simulink model "SPC_3states"  (R2019b)
settings: Solver=VariableStepAuto  StartTime=0.0  StopTime=1500  RelTol=1e-3
values from neighbouring files (symbols this model uses):
  tau1 = 15    [SmithControl.m]    (also in TimeDelayParameters.m; positivity_matrix.m)
  tau2 = 20    [SmithControl.m]    (also in TimeDelayParameters.m = 30; positivity_matrix.m = 30)
  th1 = 0.85    [AP_TimeDelay.m]    (also in SmithControl.m; TimeDelayParameters.m = 0.32; positivity_matrix.m; rscale.m)
  th2 = 50    [AP_TimeDelay.m]    (also in SmithControl.m; TimeDelayParameters.m; positivity_matrix.m; rscale.m)
  th3 = 60    [AP_TimeDelay.m]    (also in SmithControl.m; TimeDelayParameters.m = 70; positivity_matrix.m; rscale.m)
  th4 = 5    [AP_TimeDelay.m]    (also in SmithControl.m; TimeDelayParameters.m = 2.7; positivity_matrix.m; rscale.m)
  th5 = 20    [AP_TimeDelay.m]    (also in SmithControl.m; TimeDelayParameters.m = 22; positivity_matrix.m; rscale.m)
settings Model: Creator=akshita_jain  LastModifiedBy=akshita_jain

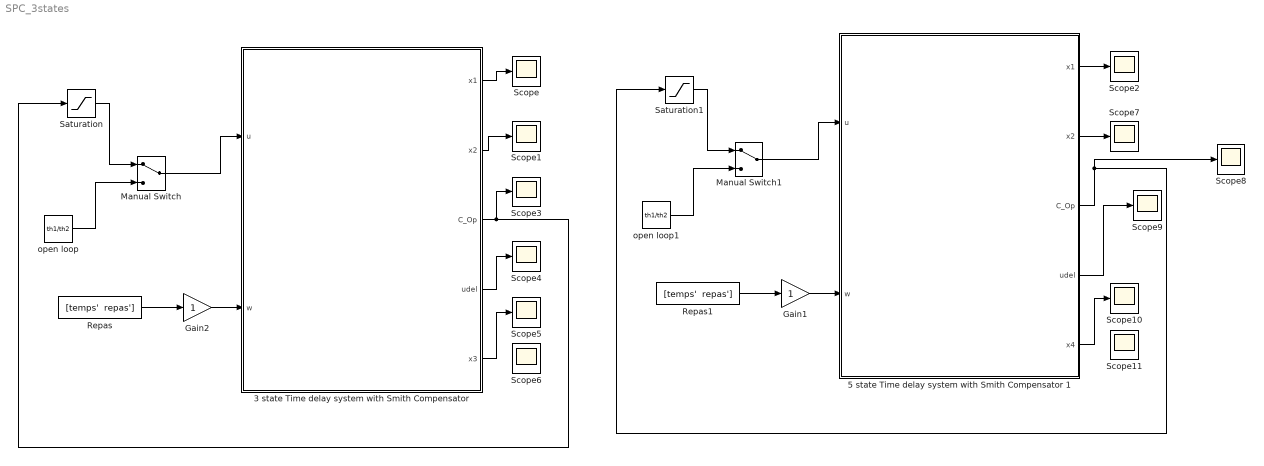
== system SPC_3states ==
  "3 state Time delay system with Smith Compensator " : Subsystem
  5 state Time delay system with Smith Compensator 1 : Subsystem
  Gain1 : Gain
  Gain2 : Gain
  Manual Switch : ManualSwitch
  Manual Switch1 : ManualSwitch
  Repas : FromWorkspace  VariableName="[temps'  repas']"  SampleTime=0
  Repas1 : FromWorkspace  VariableName="[temps'  repas']"  SampleTime=0
  Saturation : Saturate  UpperLimit=2  LowerLimit=0
  Saturation1 : Saturate  UpperLimit=2  LowerLimit=0
  Scope{,1..11} (12 alike) : Scope
  open loop : Constant  Value=th1/th2
  open loop1 : Constant  Value=th1/th2
  wires:
  "3 state Time delay system with Smith Compensator "/1(x1) -> Scope/1
  "3 state Time delay system with Smith Compensator "/3(C_Op) -> Scope3/1, Saturation/1
  "3 state Time delay system with Smith Compensator "/4(udel) -> Scope4/1
  "3 state Time delay system with Smith Compensator "/2(x2) -> Scope1/1
  Gain2/1 -> "3 state Time delay system with Smith Compensator "/2(w)
  Manual Switch/1 -> "3 state Time delay system with Smith Compensator "/1(u)
  Repas/1 -> Gain2/1
  open loop/1 -> Manual Switch/2
  Saturation/1 -> Manual Switch/1
  "3 state Time delay system with Smith Compensator "/5(x3) -> Scope5/1
  5 state Time delay system with Smith Compensator 1/1(x1) -> Scope2/1
  5 state Time delay system with Smith Compensator 1/4(udel) -> Scope9/1
  5 state Time delay system with Smith Compensator 1/2(x2) -> Scope7/1
  Gain1/1 -> 5 state Time delay system with Smith Compensator 1/2(w)
  Manual Switch1/1 -> 5 state Time delay system with Smith Compensator 1/1(u)
  open loop1/1 -> Manual Switch1/2
  Saturation1/1 -> Manual Switch1/1
  Repas1/1 -> Gain1/1
  5 state Time delay system with Smith Compensator 1/5(x4) -> Scope10/1
  5 state Time delay system with Smith Compensator 1/3(C_Op) -> Scope8/1, Saturation1/1

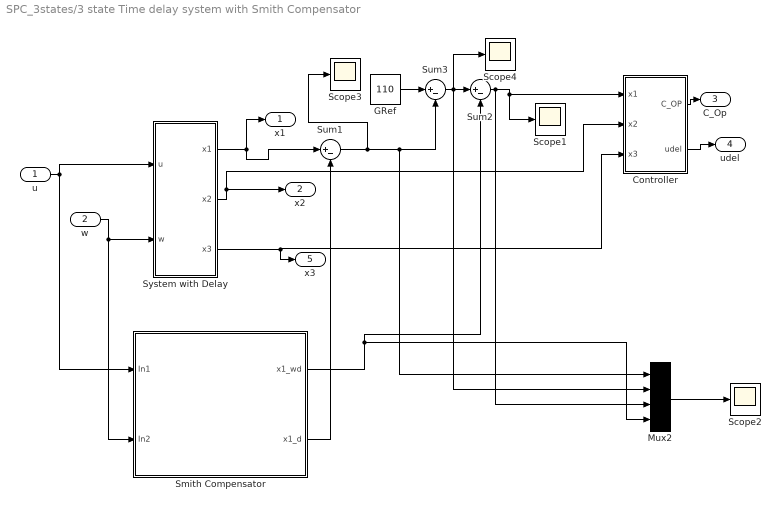
== system SPC_3states/3 state Time delay system with Smith Compensator  ==
  u : Inport
  w : Inport  Port=2
  "Controller " : Subsystem
  GRef : Constant  Value=110
  Mux2 : Mux
  Scope{1..4} (4 alike) : Scope
  Smith Compensator : Subsystem
  Sum1 : Sum  Inputs=|+-
  Sum2 : Sum  Inputs=|+-
  Sum3 : Sum  Inputs=|+-
  System with Delay : Subsystem
  x1 : Outport
  x2 : Outport  Port=2
  C_Op : Outport  Port=3
  udel : Outport  Port=4
  x3 : Outport  Port=5
  wires:
  u/1 -> Smith Compensator/1(In1), System with Delay/1(u)
  w/1 -> Smith Compensator/2(In2), System with Delay/2(w)
  System with Delay/1(x1) -> x1/1, Sum1/1
  Smith Compensator/2(x1_d) -> Sum1/2
  Sum1/1 -> Scope3/1, Mux2/1, Sum3/2
  Smith Compensator/1(x1_wd) -> Sum2/2, Mux2/4
  Sum2/1 -> Mux2/3, Scope1/1, "Controller "/1(x1)
  GRef/1 -> Sum3/1
  System with Delay/2(x2) -> "Controller "/2(x2), x2/1
  "Controller "/1(C_OP) -> C_Op/1
  "Controller "/2(udel) -> udel/1
  Mux2/1 -> Scope2/1
  Sum3/1 -> Scope4/1, Mux2/2, Sum2/1
  System with Delay/3(x3) -> "Controller "/3(x3), x3/1

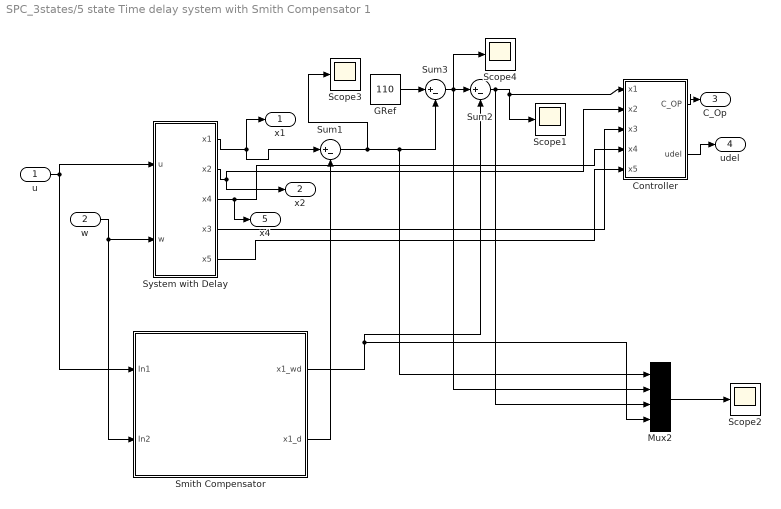
== system SPC_3states/5 state Time delay system with Smith Compensator 1 ==
  u : Inport
  w : Inport  Port=2
  "Controller " : Subsystem
  GRef : Constant  Value=110
  Mux2 : Mux
  Scope{1..4} (4 alike) : Scope
  Smith Compensator : Subsystem
  Sum1 : Sum  Inputs=|+-
  Sum2 : Sum  Inputs=|+-
  Sum3 : Sum  Inputs=|+-
  System with Delay : Subsystem
  x1 : Outport
  x2 : Outport  Port=2
  C_Op : Outport  Port=3
  udel : Outport  Port=4
  x4 : Outport  Port=5
  wires:
  u/1 -> Smith Compensator/1(In1), System with Delay/1(u)
  w/1 -> Smith Compensator/2(In2), System with Delay/2(w)
  System with Delay/1(x1) -> x1/1, Sum1/1
  Smith Compensator/2(x1_d) -> Sum1/2
  Sum1/1 -> Scope3/1, Mux2/1, Sum3/2
  Smith Compensator/1(x1_wd) -> Sum2/2, Mux2/4
  Sum2/1 -> Mux2/3, Scope1/1, "Controller "/1(x1)
  GRef/1 -> Sum3/1
  System with Delay/2(x2) -> x2/1, "Controller "/2(x2)
  "Controller "/1(C_OP) -> C_Op/1
  "Controller "/2(udel) -> udel/1
  Mux2/1 -> Scope2/1
  Sum3/1 -> Scope4/1, Mux2/2, Sum2/1
  System with Delay/4(x3) -> "Controller "/3(x3)
  System with Delay/3(x4) -> x4/1, "Controller "/4(x4)
  System with Delay/5(x5) -> "Controller "/5(x5)

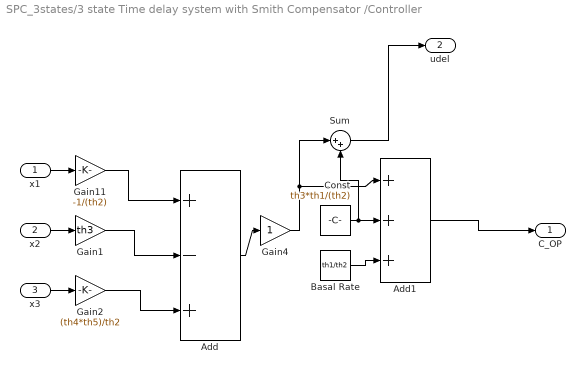
== system SPC_3states/3 state Time delay system with Smith Compensator /Controller  ==
  x1 : Inport
  x2 : Inport  Port=2
  x3 : Inport  Port=3
  Add : Sum  Inputs=+-+
  Add1 : Sum  Inputs=+++
  Basal Rate : Constant  Value=th1/th2  VectorParams1D=off
  Const : Constant  Value=th3*th1/(th2)  VectorParams1D=off
  Gain1 : Gain  Gain=th3
  Gain11 : Gain  Gain=-1/(th2)
  Gain2 : Gain  Gain=(th4*th5)/th2
  Gain4 : Gain
  Sum : Sum  Inputs=|++
  C_OP : Outport
  udel : Outport  Port=2
  wires:
  x1/1 -> Gain11/1
  x2/1 -> Gain1/1
  x3/1 -> Gain2/1
  Gain11/1 -> Add/1
  Gain1/1 -> Add/2
  Gain2/1 -> Add/3
  Add/1 -> Gain4/1
  Const/1 -> Add1/2, Sum/2
  Basal Rate/1 -> Add1/3
  Add1/1 -> C_OP/1
  Sum/1 -> udel/1
  Gain4/1 -> Sum/1, Add1/1

== system SPC_3states/3 state Time delay system with Smith Compensator /Smith Compensator ==
  In1 : Inport
  In2 : Inport  Port=2
  Scope1 : Scope
  Scope2 : Scope
  System with Delay1 : Subsystem
  System without Delay : Subsystem
  x1_wd : Outport
  x1_d : Outport  Port=2
  wires:
  System without Delay/2(Scope) -> Scope1/1
  System with Delay1/1(x1_d) -> x1_d/1
  System without Delay/1(x1_wd) -> x1_wd/1
  System with Delay1/2(Scope) -> Scope2/1
  In2/1 -> System with Delay1/2(w), System without Delay/2(w)
  In1/1 -> System with Delay1/1(u), System without Delay/1(u)

== system SPC_3states/3 state Time delay system with Smith Compensator /System with Delay ==
  u : Inport
  w : Inport  Port=2
  CHO : Subsystem
  Glucose : Subsystem
  Insulin Plasma : Subsystem
  x1 : Outport
  x2 : Outport  Port=2
  x3 : Outport  Port=3
  wires:
  Glucose/1(x1) -> x1/1
  w/1 -> CHO/1(w)
  Insulin Plasma/1(x2) -> Glucose/1(x2), x2/1
  u/1 -> Insulin Plasma/1(u)
  CHO/1(x3) -> x3/1, Glucose/2(x3)

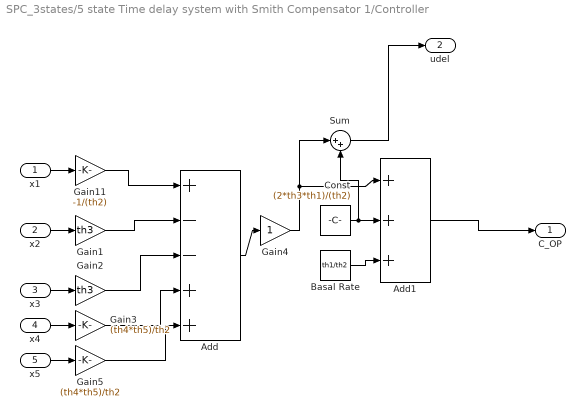
== system SPC_3states/5 state Time delay system with Smith Compensator 1/Controller  ==
  x1 : Inport
  x2 : Inport  Port=2
  x3 : Inport  Port=3
  x4 : Inport  Port=4
  x5 : Inport  Port=5
  Add : Sum  Inputs=+--++
  Add1 : Sum  Inputs=+++
  Basal Rate : Constant  Value=th1/th2  VectorParams1D=off
  Const : Constant  Value=(2*th3*th1)/(th2)  VectorParams1D=off
  Gain1 : Gain  Gain=th3
  Gain11 : Gain  Gain=-1/(th2)
  Gain2 : Gain  Gain=th3
  Gain3 : Gain  Gain=(th4*th5)/th2
  Gain4 : Gain
  Gain5 : Gain  Gain=(th4*th5)/th2
  Sum : Sum  Inputs=|++
  C_OP : Outport
  udel : Outport  Port=2
  wires:
  x1/1 -> Gain11/1
  x2/1 -> Gain1/1
  x3/1 -> Gain2/1
  Gain11/1 -> Add/1
  Gain1/1 -> Add/2
  Gain2/1 -> Add/3
  Add/1 -> Gain4/1
  Const/1 -> Add1/2, Sum/2
  Basal Rate/1 -> Add1/3
  Add1/1 -> C_OP/1
  Sum/1 -> udel/1
  Gain4/1 -> Sum/1, Add1/1
  x4/1 -> Gain3/1
  x5/1 -> Gain5/1
  Gain3/1 -> Add/4
  Gain5/1 -> Add/5

== system SPC_3states/5 state Time delay system with Smith Compensator 1/Smith Compensator ==
  In1 : Inport
  In2 : Inport  Port=2
  Scope1 : Scope
  Scope2 : Scope
  System with Delay1 : Subsystem
  System without Delay : Subsystem
  x1_wd : Outport
  x1_d : Outport  Port=2
  wires:
  System without Delay/2(Scope) -> Scope1/1
  System with Delay1/1(x1_d) -> x1_d/1
  System without Delay/1(x1_wd) -> x1_wd/1
  System with Delay1/2(Scope) -> Scope2/1
  In2/1 -> System with Delay1/2(w), System without Delay/2(w)
  In1/1 -> System with Delay1/1(u), System without Delay/1(u)

== system SPC_3states/5 state Time delay system with Smith Compensator 1/System with Delay ==
  u : Inport
  w : Inport  Port=2
  CHO : Subsystem
  Glucose : Subsystem
  Insulin Plasma : Subsystem
  x1 : Outport
  x2 : Outport  Port=2
  x4 : Outport  Port=3
  x3 : Outport  Port=4
  x5 : Outport  Port=5
  wires:
  Glucose/1(x1) -> x1/1
  w/1 -> CHO/1(w1)
  Insulin Plasma/1(x2) -> Glucose/1(x2), x2/1
  u/1 -> Insulin Plasma/1(u1)
  CHO/1(x4) -> Glucose/2(x4), x4/1
  Insulin Plasma/2(x3) -> x3/1
  CHO/2(x5) -> x5/1

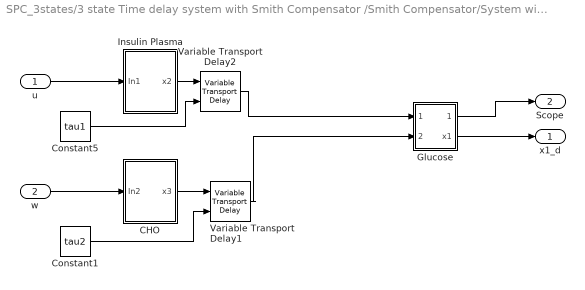
== system SPC_3states/3 state Time delay system with Smith Compensator /Smith Compensator/System with Delay1 ==
  u : Inport
  w : Inport  Port=2
  CHO : Subsystem
  Constant1 : Constant  Value=tau2
  Constant5 : Constant  Value=tau1
  Glucose : Subsystem
  Insulin Plasma : Subsystem
  Variable Transport Delay1 : VariableTransportDelay  VariableDelayType=Variable transport delay  MaximumDelay=30
  Variable Transport Delay2 : VariableTransportDelay  VariableDelayType=Variable transport delay  MaximumDelay=20  InitialOutput=th1/th2
  x1_d : Outport
  Scope : Outport  Port=2
  wires:
  Glucose/2(x1) -> x1_d/1
  w/1 -> CHO/1(In2)
  u/1 -> Insulin Plasma/1(In1)
  Variable Transport Delay2/1 -> Glucose/1(In1)
  Insulin Plasma/1(x2) -> Variable Transport Delay2/1
  Constant5/1 -> Variable Transport Delay2/2
  CHO/1(x3) -> Variable Transport Delay1/1
  Variable Transport Delay1/1 -> Glucose/2(In2)
  Constant1/1 -> Variable Transport Delay1/2
  Glucose/1(Out1) -> Scope/1

== system SPC_3states/3 state Time delay system with Smith Compensator /Smith Compensator/System without Delay ==
  u : Inport
  w : Inport  Port=2
  CHO : Subsystem
  Glucose : Subsystem
  Insulin Plasma : Subsystem
  x1_wd : Outport
  Scope : Outport  Port=2
  wires:
  Glucose/2(x1) -> x1_wd/1
  w/1 -> CHO/1(In2)
  Insulin Plasma/1(x2) -> Glucose/1(In1)
  u/1 -> Insulin Plasma/1(In1)
  Glucose/1(Out1) -> Scope/1
  CHO/1(x3) -> Glucose/2(In2)

== system SPC_3states/3 state Time delay system with Smith Compensator /System with Delay/CHO ==
  w : Inport
  Add1 : Sum  Inputs=-+
  Constant1 : Constant  Value=tau2  VectorParams1D=off
  Gain1 : Gain  Gain=1/th5
  Gain2 : Gain  Gain=1/th5
  Integrator1 : Integrator  ZeroCross=off
  Variable Transport Delay1 : VariableTransportDelay  VariableDelayType=Variable transport delay  MaximumDelay=35
  x3 : Outport
  wires:
  Variable Transport Delay1/1 -> Gain1/1
  Add1/1 -> Integrator1/1
  Constant1/1 -> Variable Transport Delay1/2
  Gain2/1 -> Add1/1
  Gain1/1 -> Add1/2
  Integrator1/1 -> x3/1, Gain2/1
  w/1 -> Variable Transport Delay1/1

== system SPC_3states/3 state Time delay system with Smith Compensator /System with Delay/Glucose ==
  x2 : Inport
  x3 : Inport  Port=2
  Add4 : Sum  Inputs=+-+
  Constant4 : Constant  Value=th1  VectorParams1D=off
  Gain2 : Gain  Gain=th2
  Gain4 : Gain  Gain=th4
  Integrator4 : Integrator  InitialCondition=110  ZeroCross=off
  x1 : Outport
  wires:
  Gain2/1 -> Add4/2
  x3/1 -> Gain4/1
  x2/1 -> Gain2/1
  Add4/1 -> Integrator4/1
  Constant4/1 -> Add4/1
  Integrator4/1 -> x1/1
  Gain4/1 -> Add4/3

== system SPC_3states/3 state Time delay system with Smith Compensator /System with Delay/Insulin Plasma ==
  u : Inport
  Add1 : Sum  Inputs=-+
  Constant1 : Constant  Value=tau1
  Gain1 : Gain  Gain=1/th3
  Gain2 : Gain  Gain=1/th3
  Integrator1 : Integrator  InitialCondition=th1/th2  ZeroCross=off
  Variable Transport Delay1 : VariableTransportDelay  VariableDelayType=Variable transport delay  MaximumDelay=20  InitialOutput=th1/th2
  x2 : Outport
  wires:
  Constant1/1 -> Variable Transport Delay1/2
  Add1/1 -> Integrator1/1
  Integrator1/1 -> x2/1, Gain2/1
  Gain1/1 -> Add1/2
  Gain2/1 -> Add1/1
  Variable Transport Delay1/1 -> Gain1/1
  u/1 -> Variable Transport Delay1/1

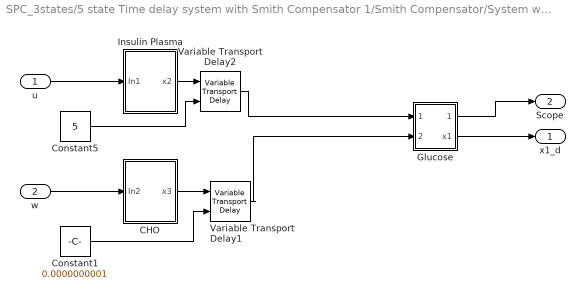
== system SPC_3states/5 state Time delay system with Smith Compensator 1/Smith Compensator/System with Delay1 ==
  u : Inport
  w : Inport  Port=2
  CHO : Subsystem
  Constant1 : Constant  Value=0.0000000001
  Constant5 : Constant  Value=5
  Glucose : Subsystem
  Insulin Plasma : Subsystem
  Variable Transport Delay1 : VariableTransportDelay  VariableDelayType=Variable transport delay  MaximumDelay=30
  Variable Transport Delay2 : VariableTransportDelay  VariableDelayType=Variable transport delay  MaximumDelay=20  InitialOutput=th1/th2
  x1_d : Outport
  Scope : Outport  Port=2
  wires:
  Glucose/2(x1) -> x1_d/1
  w/1 -> CHO/1(In2)
  u/1 -> Insulin Plasma/1(In1)
  Variable Transport Delay2/1 -> Glucose/1(In1)
  Insulin Plasma/1(x2) -> Variable Transport Delay2/1
  Constant5/1 -> Variable Transport Delay2/2
  CHO/1(x3) -> Variable Transport Delay1/1
  Variable Transport Delay1/1 -> Glucose/2(In2)
  Constant1/1 -> Variable Transport Delay1/2
  Glucose/1(Out1) -> Scope/1

== system SPC_3states/5 state Time delay system with Smith Compensator 1/Smith Compensator/System without Delay ==
  u : Inport
  w : Inport  Port=2
  CHO : Subsystem
  Glucose : Subsystem
  Insulin Plasma : Subsystem
  x1_wd : Outport
  Scope : Outport  Port=2
  wires:
  Glucose/2(x1) -> x1_wd/1
  w/1 -> CHO/1(In2)
  Insulin Plasma/1(x2) -> Glucose/1(In1)
  u/1 -> Insulin Plasma/1(In1)
  Glucose/1(Out1) -> Scope/1
  CHO/1(x3) -> Glucose/2(In2)

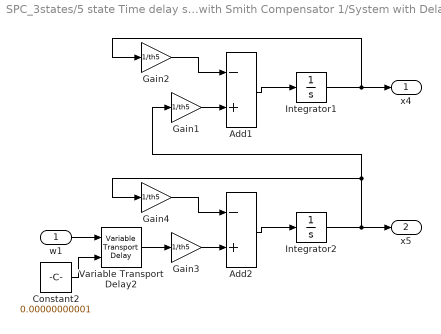
== system SPC_3states/5 state Time delay system with Smith Compensator 1/System with Delay/CHO ==
  w1 : Inport
  Add1 : Sum  Inputs=-+
  Add2 : Sum  Inputs=-+
  Constant2 : Constant  Value=0.00000000001  VectorParams1D=off
  Gain{1..4} (4 alike) : Gain  Gain=1/th5
  Integrator1 : Integrator  ZeroCross=off
  Integrator2 : Integrator  ZeroCross=off
  Variable Transport Delay2 : VariableTransportDelay  VariableDelayType=Variable transport delay  MaximumDelay=35
  x4 : Outport
  x5 : Outport  Port=2
  wires:
  Add1/1 -> Integrator1/1
  Gain2/1 -> Add1/1
  Gain1/1 -> Add1/2
  Integrator1/1 -> x4/1, Gain2/1
  Gain3/1 -> Add2/2
  Integrator2/1 -> x5/1, Gain1/1, Gain4/1
  w1/1 -> Variable Transport Delay2/1
  Variable Transport Delay2/1 -> Gain3/1
  Constant2/1 -> Variable Transport Delay2/2
  Add2/1 -> Integrator2/1
  Gain4/1 -> Add2/1

== system SPC_3states/5 state Time delay system with Smith Compensator 1/System with Delay/Glucose ==
  x2 : Inport
  x4 : Inport  Port=2
  Add4 : Sum  Inputs=+-+
  Constant4 : Constant  Value=th1  VectorParams1D=off
  Gain2 : Gain  Gain=th2
  Gain4 : Gain  Gain=th4
  Integrator4 : Integrator  InitialCondition=110  ZeroCross=off
  x1 : Outport
  wires:
  Gain2/1 -> Add4/2
  x4/1 -> Gain4/1
  x2/1 -> Gain2/1
  Add4/1 -> Integrator4/1
  Constant4/1 -> Add4/1
  Integrator4/1 -> x1/1
  Gain4/1 -> Add4/3

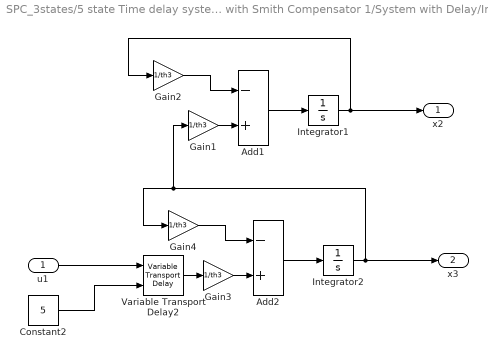
== system SPC_3states/5 state Time delay system with Smith Compensator 1/System with Delay/Insulin Plasma ==
  u1 : Inport
  Add1 : Sum  Inputs=-+
  Add2 : Sum  Inputs=-+
  Constant2 : Constant  Value=5
  Gain{1..4} (4 alike) : Gain  Gain=1/th3
  Integrator1 : Integrator  InitialCondition=th1/th2  ZeroCross=off
  Integrator2 : Integrator  InitialCondition=th1/th2  ZeroCross=off
  Variable Transport Delay2 : VariableTransportDelay  VariableDelayType=Variable transport delay  MaximumDelay=20  InitialOutput=th1/th2
  x2 : Outport
  x3 : Outport  Port=2
  wires:
  Add1/1 -> Integrator1/1
  Integrator1/1 -> x2/1, Gain2/1
  Gain1/1 -> Add1/2
  Gain2/1 -> Add1/1
  Add2/1 -> Integrator2/1
  u1/1 -> Variable Transport Delay2/1
  Variable Transport Delay2/1 -> Gain3/1
  Gain4/1 -> Add2/1
  Constant2/1 -> Variable Transport Delay2/2
  Gain3/1 -> Add2/2
  Integrator2/1 -> x3/1, Gain1/1, Gain4/1

== system SPC_3states/3 state Time delay system with Smith Compensator /Smith Compensator/System with Delay1/CHO ==
  In2 : Inport
  Add1 : Sum  Inputs=-+
  Gain1 : Gain  Gain=1/th5
  Gain2 : Gain  Gain=1/th5
  Integrator1 : Integrator  ZeroCross=off
  x3 : Outport
  wires:
  Add1/1 -> Integrator1/1
  Gain2/1 -> Add1/1
  Integrator1/1 -> x3/1, Gain2/1
  Gain1/1 -> Add1/2
  In2/1 -> Gain1/1

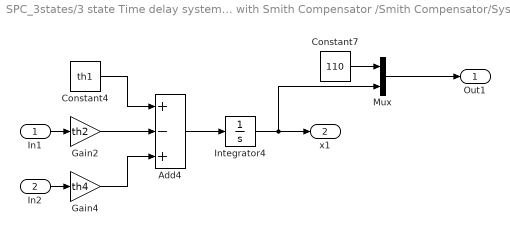
== system SPC_3states/3 state Time delay system with Smith Compensator /Smith Compensator/System with Delay1/Glucose ==
  In1 : Inport
  In2 : Inport  Port=2
  Add4 : Sum  Inputs=+-+
  Constant4 : Constant  Value=th1  VectorParams1D=off
  Constant7 : Constant  Value=110  VectorParams1D=off
  Gain2 : Gain  Gain=th2
  Gain4 : Gain  Gain=th4
  Integrator4 : Integrator  InitialCondition=110  ZeroCross=off
  Mux : Mux  Inputs=2
  Out1 : Outport
  x1 : Outport  Port=2
  wires:
  Gain2/1 -> Add4/2
  In2/1 -> Gain4/1
  In1/1 -> Gain2/1
  Mux/1 -> Out1/1
  Add4/1 -> Integrator4/1
  Constant4/1 -> Add4/1
  Integrator4/1 -> x1/1, Mux/2
  Gain4/1 -> Add4/3
  Constant7/1 -> Mux/1

== system SPC_3states/3 state Time delay system with Smith Compensator /Smith Compensator/System with Delay1/Insulin Plasma ==
  In1 : Inport
  Add1 : Sum  Inputs=-+
  Gain1 : Gain  Gain=1/th3
  Gain2 : Gain  Gain=1/th3
  Integrator1 : Integrator  InitialCondition=th1/th2  ZeroCross=off
  x2 : Outport
  wires:
  Gain1/1 -> Add1/2
  Gain2/1 -> Add1/1
  Add1/1 -> Integrator1/1
  Integrator1/1 -> x2/1, Gain2/1
  In1/1 -> Gain1/1

== system SPC_3states/3 state Time delay system with Smith Compensator /Smith Compensator/System without Delay/CHO ==
  In2 : Inport
  Add1 : Sum  Inputs=-+
  Gain1 : Gain  Gain=1/th5
  Gain2 : Gain  Gain=1/th5
  Integrator1 : Integrator  ZeroCross=off
  x3 : Outport
  wires:
  Add1/1 -> Integrator1/1
  Gain2/1 -> Add1/1
  Gain1/1 -> Add1/2
  Integrator1/1 -> x3/1, Gain2/1
  In2/1 -> Gain1/1

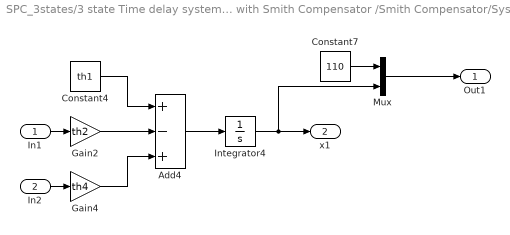
== system SPC_3states/3 state Time delay system with Smith Compensator /Smith Compensator/System without Delay/Glucose ==
  In1 : Inport
  In2 : Inport  Port=2
  Add4 : Sum  Inputs=+-+
  Constant4 : Constant  Value=th1  VectorParams1D=off
  Constant7 : Constant  Value=110  VectorParams1D=off
  Gain2 : Gain  Gain=th2
  Gain4 : Gain  Gain=th4
  Integrator4 : Integrator  InitialCondition=110  ZeroCross=off
  Mux : Mux  Inputs=2
  Out1 : Outport
  x1 : Outport  Port=2
  wires:
  Gain2/1 -> Add4/2
  In2/1 -> Gain4/1
  In1/1 -> Gain2/1
  Mux/1 -> Out1/1
  Add4/1 -> Integrator4/1
  Constant4/1 -> Add4/1
  Integrator4/1 -> x1/1, Mux/2
  Gain4/1 -> Add4/3
  Constant7/1 -> Mux/1

== system SPC_3states/3 state Time delay system with Smith Compensator /Smith Compensator/System without Delay/Insulin Plasma ==
  In1 : Inport
  Add1 : Sum  Inputs=-+
  Gain1 : Gain  Gain=1/th3
  Gain2 : Gain  Gain=1/th3
  Integrator1 : Integrator  InitialCondition=th1/th2  ZeroCross=off
  x2 : Outport
  wires:
  Add1/1 -> Integrator1/1
  Gain1/1 -> Add1/2
  Gain2/1 -> Add1/1
  Integrator1/1 -> x2/1, Gain2/1
  In1/1 -> Gain1/1

== system SPC_3states/5 state Time delay system with Smith Compensator 1/Smith Compensator/System with Delay1/CHO ==
  In2 : Inport
  Add1 : Sum  Inputs=-+
  Gain1 : Gain  Gain=1/th5
  Gain2 : Gain  Gain=1/th5
  Integrator1 : Integrator  ZeroCross=off
  x3 : Outport
  wires:
  Add1/1 -> Integrator1/1
  Gain2/1 -> Add1/1
  Integrator1/1 -> x3/1, Gain2/1
  Gain1/1 -> Add1/2
  In2/1 -> Gain1/1

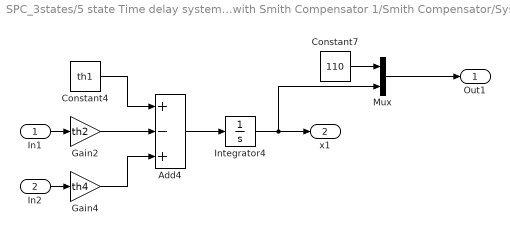
== system SPC_3states/5 state Time delay system with Smith Compensator 1/Smith Compensator/System with Delay1/Glucose ==
  In1 : Inport
  In2 : Inport  Port=2
  Add4 : Sum  Inputs=+-+
  Constant4 : Constant  Value=th1  VectorParams1D=off
  Constant7 : Constant  Value=110  VectorParams1D=off
  Gain2 : Gain  Gain=th2
  Gain4 : Gain  Gain=th4
  Integrator4 : Integrator  InitialCondition=110  ZeroCross=off
  Mux : Mux  Inputs=2
  Out1 : Outport
  x1 : Outport  Port=2
  wires:
  Gain2/1 -> Add4/2
  In2/1 -> Gain4/1
  In1/1 -> Gain2/1
  Mux/1 -> Out1/1
  Add4/1 -> Integrator4/1
  Constant4/1 -> Add4/1
  Integrator4/1 -> x1/1, Mux/2
  Gain4/1 -> Add4/3
  Constant7/1 -> Mux/1

== system SPC_3states/5 state Time delay system with Smith Compensator 1/Smith Compensator/System with Delay1/Insulin Plasma ==
  In1 : Inport
  Add1 : Sum  Inputs=-+
  Gain1 : Gain  Gain=1/th3
  Gain2 : Gain  Gain=1/th3
  Integrator1 : Integrator  InitialCondition=th1/th2  ZeroCross=off
  x2 : Outport
  wires:
  Gain1/1 -> Add1/2
  Gain2/1 -> Add1/1
  Add1/1 -> Integrator1/1
  Integrator1/1 -> x2/1, Gain2/1
  In1/1 -> Gain1/1

== system SPC_3states/5 state Time delay system with Smith Compensator 1/Smith Compensator/System without Delay/CHO ==
  In2 : Inport
  Add1 : Sum  Inputs=-+
  Gain1 : Gain  Gain=1/th5
  Gain2 : Gain  Gain=1/th5
  Integrator1 : Integrator  ZeroCross=off
  x3 : Outport
  wires:
  Add1/1 -> Integrator1/1
  Gain2/1 -> Add1/1
  Gain1/1 -> Add1/2
  Integrator1/1 -> x3/1, Gain2/1
  In2/1 -> Gain1/1

== system SPC_3states/5 state Time delay system with Smith Compensator 1/Smith Compensator/System without Delay/Glucose ==
  In1 : Inport
  In2 : Inport  Port=2
  Add4 : Sum  Inputs=+-+
  Constant4 : Constant  Value=th1  VectorParams1D=off
  Constant7 : Constant  Value=110  VectorParams1D=off
  Gain2 : Gain  Gain=th2
  Gain4 : Gain  Gain=th4
  Integrator4 : Integrator  InitialCondition=110  ZeroCross=off
  Mux : Mux  Inputs=2
  Out1 : Outport
  x1 : Outport  Port=2
  wires:
  Gain2/1 -> Add4/2
  In2/1 -> Gain4/1
  In1/1 -> Gain2/1
  Mux/1 -> Out1/1
  Add4/1 -> Integrator4/1
  Constant4/1 -> Add4/1
  Integrator4/1 -> x1/1, Mux/2
  Gain4/1 -> Add4/3
  Constant7/1 -> Mux/1

== system SPC_3states/5 state Time delay system with Smith Compensator 1/Smith Compensator/System without Delay/Insulin Plasma ==
  In1 : Inport
  Add1 : Sum  Inputs=-+
  Gain1 : Gain  Gain=1/th3
  Gain2 : Gain  Gain=1/th3
  Integrator1 : Integrator  InitialCondition=th1/th2  ZeroCross=off
  x2 : Outport
  wires:
  Add1/1 -> Integrator1/1
  Gain1/1 -> Add1/2
  Gain2/1 -> Add1/1
  Integrator1/1 -> x2/1, Gain2/1
  In1/1 -> Gain1/1
